simulink model "FSK"  (R2019b)
settings: Solver=VariableStepAuto  StartTime=0.0  StopTime=10.0  RelTol=1e-3
libraries: commfilt2 x2, commrandsrc3 x1
settings Model: Creator=DELL  LastModifiedBy=DELL

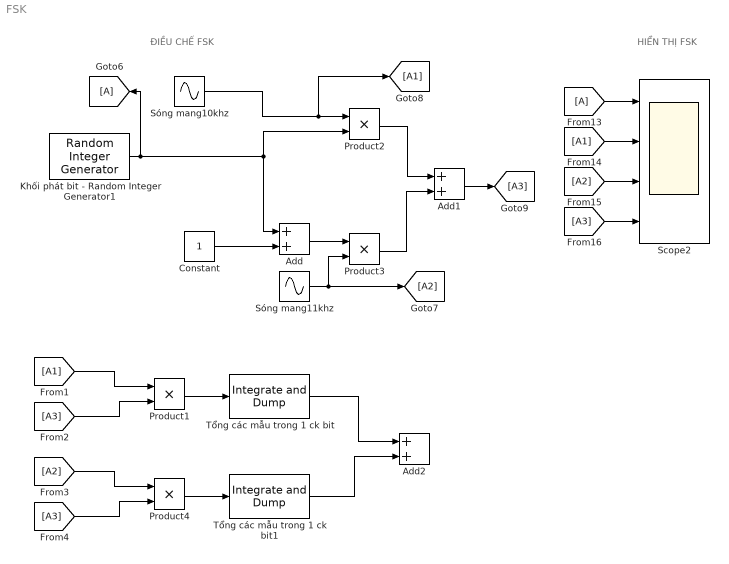
== system FSK ==
  note: HIỂN THỊ FSK
  note: ĐIỀU CHẾ FSK
  Add : Sum
  Add1 : Sum
  Add2 : Sum
  Constant : Constant
  Khối phát bit - Random Integer Generator1 : commrandsrc3/Random Integer Generator  SetSize=2  SeedSource=Auto  Seed=0  SampleTime=1/1000  SamplesPerFrame=1  OutputDataType=double  SimulateUsing=Interpreted execution
      settings: SourceProductName=Communications Toolbox
  Product{1..4} (4 alike) : Product
  Scope2 : Scope  NumInputPorts=4
  Sóng mang10khz : Sin  Frequency=2*pi*10000  SampleTime=1/100000
  Sóng mang11khz : Sin  Frequency=2*pi*11000  SampleTime=1/100000
  Tổng các mẫu trong 1 ck bit : commfilt2/Integrate and Dump  obssamples=8  offsetsamples=0  nodump=off  roundingMode=Floor  overflowMode=off  outputDataTypeStr=Inherit: Same as accumulator  outputLastDataTypeStr=Inherit: Same as accumulator
      settings: SourceProductName=Communications Toolbox
  Tổng các mẫu trong 1 ck bit1 : commfilt2/Integrate and Dump  obssamples=8  offsetsamples=0  nodump=off  roundingMode=Floor  overflowMode=off  outputDataTypeStr=Inherit: Same as accumulator  outputLastDataTypeStr=Inherit: Same as accumulator
      settings: SourceProductName=Communications Toolbox
  wires:
  Product3/1 -> Add1/2
  Product2/1 -> Add1/1
  Add/1 -> Product3/1
  Khối phát bit - Random Integer Generator1/1 -> Add/1, Product2/2, [A]
  Sóng mang11khz/1 -> [A2], Product3/2
  Add1/1 -> [A3]
  Constant/1 -> Add/2
  Sóng mang10khz/1 -> [A1], Product2/1
  [A1] -> Scope2/2
  [A3] -> Scope2/4
  [A2] -> Scope2/3
  [A] -> Scope2/1
  Product4/1 -> Tổng các mẫu trong 1 ck bit1/1
  Product1/1 -> Tổng các mẫu trong 1 ck bit/1
  [A3] -> Product1/2
  [A3] -> Product4/2
  [A2] -> Product4/1
  Tổng các mẫu trong 1 ck bit1/1 -> Add2/2
  [A1] -> Product1/1
  Tổng các mẫu trong 1 ck bit/1 -> Add2/1
